simulink model "StewartPlatformSimulation"  (R2022b)
settings: Solver=VariableStepAuto  StartTime=0.0  StopTime=TF  FixedStep=stepSize  RelTol=1e-3
values from neighbouring files (symbols this model uses):
  a = s * armLegRatio    [StewartPlatformEqs.m]    (also in StewartPlatformEqs_JointAngles.m; StewartPlatformEqs_alpha.m; findRangeOfMotion_disturbance.m = 2; findh0.m)
  A0 = zeros(3,6)    [runSimulation.m]
  alpha0 = ones(1,6) * servoCalc(P_default(:,1),b(:,1),sqrt(l0_squared),s,a,beta(1))    [StewartPlatformEqs.m]    (also in StewartPlatformEqs_JointAngles.m; StewartPlatformEqs_alpha.m; runSimulation.m = alpha0')
  alpha_max = servoCenterOfRange + servoMotorRange/2    [StewartPlatformEqs.m]    (also in StewartPlatformEqs_JointAngles.m; StewartPlatformEqs_alpha.m; runSimulation.m)
  alpha_min = servoCenterOfRange - servoMotorRange/2    [StewartPlatformEqs.m]    (also in StewartPlatformEqs_JointAngles.m; StewartPlatformEqs_alpha.m; runSimulation.m)
  B = zeros(3,6)    [runSimulation.m]    (also in test.m = [0.996194698091746	0.996194698091746	-0.422618261740699	-0.5)
  beta = zeros(1,6)    [StewartPlatformEqs.m]    (also in StewartPlatformEqs_JointAngles.m; StewartPlatformEqs_alpha.m; runSimulation.m; test.m)
  defaultLegs = sqrt(l0_squared) .* ones(6,1)    [runSimulation.m]
  h0 = sqrt(l0_squared - (p(1,1) - b(1,1))^2 - (p(2,1) - b(2,1))^2) - p(3,1)    [StewartPlatformEqs.m]    (also in StewartPlatformEqs_JointAngles.m; StewartPlatformEqs_alpha.m; findROM_disturbance.m = platformParams.defaultHeight; findh0.m)
  l_max = s + a    [StewartPlatformEqs.m]    (also in StewartPlatformEqs_JointAngles.m; StewartPlatformEqs_alpha.m; runSimulation.m)
  P = circshift(P,[0 1])    [runSimulation.m]    (also in test.m = [0.458861149080837	0.458861149080837	0.338094609392560	-0.79)
  P_default = Tdefault + p    [StewartPlatformEqs.m]    (also in StewartPlatformEqs_JointAngles.m; StewartPlatformEqs_alpha.m; runSimulation.m = Tdefault + P)
  s = sqrt(legRestingLength^2 / (1+armLegRatio))    [StewartPlatformEqs.m]    (also in StewartPlatformEqs_JointAngles.m; StewartPlatformEqs_alpha.m; findh0.m; runSimulation.m = sqrt(restingLegLength^2 / (1+armLegRatio)))
settings Model: Creator=peter  LastModifiedBy=peter
settings DebuggingCC: UnderSpecifiedDimensionMsg=error

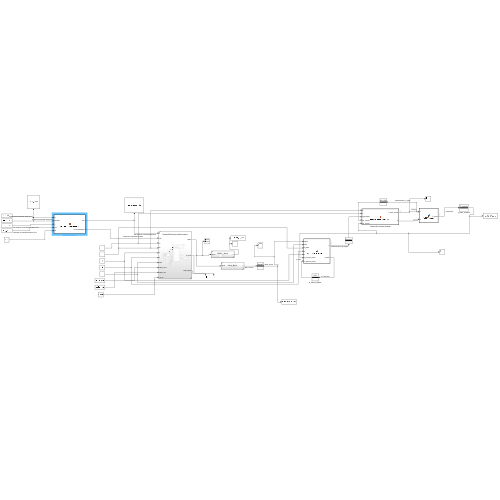
[thumbnail: Simulink's stored preview of the top-level diagram]
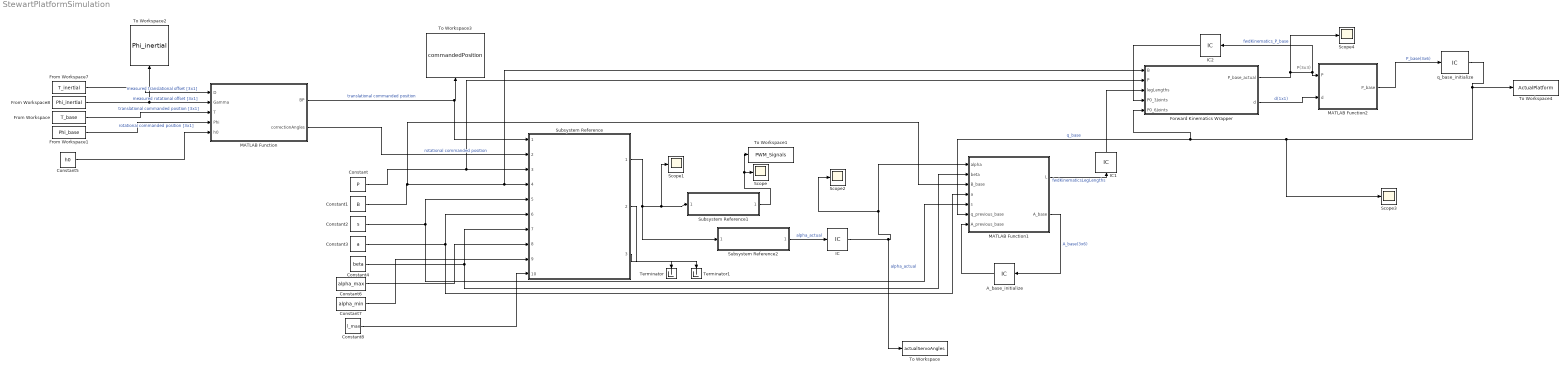
== system StewartPlatformSimulation ==
  note: P(3x3)
  A_base_initialize : InitialCondition  Value=A0
  Constant : Constant  Value=P
  Constant1 : Constant  Value=B
  Constant2 : Constant  Value=s
  Constant3 : Constant  Value=a
  Constant4 : Constant  Value=beta
  Constant5 : Constant  Value=h0
  Constant6 : Constant  Value=alpha_max
  Constant7 : Constant  Value=alpha_min
  Constant8 : Constant  Value=l_max
  Forward Kinematics Wrapper : MATLAB Function  TreatAsAtomicUnit=on
  From Workspace : FromWorkspace  VariableName=T_base
  From Workspace1 : FromWorkspace  VariableName=Phi_base
  From Workspace7 : FromWorkspace  VariableName=T_inertial
  From Workspace8 : FromWorkspace  VariableName=Phi_inertial
  IC : InitialCondition  Value=alpha0
  IC1 : InitialCondition  Value=defaultLegs
  IC2 : InitialCondition  Value=[0 0 0;0 0 0;0 0 0]
  MATLAB Function : MATLAB Function  TreatAsAtomicUnit=on
  MATLAB Function1 : MATLAB Function  TreatAsAtomicUnit=on
  MATLAB Function2 : MATLAB Function  TreatAsAtomicUnit=on
  Scope{,1..4} (5 alike) : Scope
  Subsystem Reference : Subsystem  ReferencedSubsystem=StewartPlatformInverseKinematics
  Subsystem Reference1 : Subsystem  ReferencedSubsystem=MyRio__block
  Subsystem Reference2 : Subsystem  ReferencedSubsystem=Servo_Block
  Terminator : Terminator
  Terminator1 : Terminator
  To Workspace : ToWorkspace  VariableName=actualServoAngles  SaveFormat=Timeseries  SampleTime=-1
  To Workspace1 : ToWorkspace  VariableName=PWM_Signals  SaveFormat=Timeseries  SampleTime=-1
  To Workspace2 : ToWorkspace  VariableName=Phi_inertial  SaveFormat=Timeseries  SampleTime=-1
  To Workspace3 : ToWorkspace  VariableName=commandedPosition  SaveFormat=Timeseries  SampleTime=-1
  To Workspace4 : ToWorkspace  VariableName=ActualPlatform  SaveFormat=Timeseries  SampleTime=-1
  q_base_initialize : InitialCondition  Value=P_default
  wires:
  MATLAB Function/1(BP) -> Subsystem Reference/1, To Workspace3/1  "translational commanded position"
  MATLAB Function/2(correctionAngles) -> Subsystem Reference/2  "rotational commanded position"
  Constant/1 -> Forward Kinematics Wrapper/2(P), Subsystem Reference/3
  Constant1/1 -> MATLAB Function1/3(B_base), Forward Kinematics Wrapper/1(B), Subsystem Reference/4
  Constant2/1 -> MATLAB Function1/5(s), Subsystem Reference/5
  Constant3/1 -> Subsystem Reference/6, MATLAB Function1/4(a)
  Constant4/1 -> Subsystem Reference/7, MATLAB Function1/2(beta)
  From Workspace1/1 -> MATLAB Function/4(Phi)  "rotational commanded position [3x1]"
  From Workspace/1 -> MATLAB Function/3(T)  "translational commanded position [3x1]"
  From Workspace8/1 -> MATLAB Function/2(Gamma), To Workspace2/1  "measured rotational offset [3x1]"
  From Workspace7/1 -> MATLAB Function/1(D)  "measured translational offset [3x1]"
  Subsystem Reference/1 -> Subsystem Reference2/1, Scope1/1, Subsystem Reference1/1
  Subsystem Reference1/1 -> To Workspace1/1, Scope/1
  Constant5/1 -> MATLAB Function/5(h0)
  Constant6/1 -> Subsystem Reference/8
  Constant7/1 -> Subsystem Reference/9
  Constant8/1 -> Subsystem Reference/10
  IC/1 -> To Workspace/1, Scope2/1, MATLAB Function1/1(alpha)  "alpha_actual"
  Subsystem Reference/2 -> Terminator1/1
  Subsystem Reference/3 -> Terminator/1
  MATLAB Function1/2(A_base) -> A_base_initialize/1  "A_base(3x6)"
  IC1/1 -> Forward Kinematics Wrapper/3(legLengths)
  A_base_initialize/1 -> MATLAB Function1/7(A_previous_base)
  q_base_initialize/1 -> To Workspace4/1, Scope3/1, Forward Kinematics Wrapper/5(P0_6Joints), MATLAB Function1/6(q_previous_base)  "q_base"
  Subsystem Reference2/1 -> IC/1  "alpha_actual"
  MATLAB Function2/1(P_base) -> q_base_initialize/1  "P_base(3x6)"
  Forward Kinematics Wrapper/2(d) -> MATLAB Function2/2(d)  "d(1x1)"
  Forward Kinematics Wrapper/1(P_base_actual) -> Scope4/1, IC2/1, MATLAB Function2/1(P)  "fwdKinematics_P_base"
  MATLAB Function1/1(L) -> IC1/1  "fwdKinematicsLegLengths"
  IC2/1 -> Forward Kinematics Wrapper/4(P0_3Joints)

== matlab function StewartPlatformSimulation/MATLAB Function ==
  data: D input; BP output; Gamma input; T input; Phi input; correctionAngles output; h0 input
function [BP, correctionAngles] = baseToStaticPlatformPosition(D,Gamma,T,Phi,h0)
% calculate angle offset from inertial frame
gammaX = Gamma(1) + Phi(1);
gammaY = Gamma(2) + Phi(2);
gammaZ = Gamma(3) + Phi(3);

OP = T+[0;0;h0]; % vector from origin of inertial frame (O) to origin of platform (P)

R = rotz(gammaZ)*roty(gammaY)*rotx(gammaX); % 3x3 rotation matrix

BP = D + R'*(OP - D); %BP is the base origin to platform origin vector
correctionAngles = -Gamma;
BP

== matlab function StewartPlatformSimulation/Forward Kinematics Wrapper ==
  data: B input; P_base_actual output; P input; legLengths input; d output; P0_3Joints input; P0_6Joints input
function [P_base_actual,d]  = forwardKinematicsWrapper(B,P,legLengths, P0_3Joints, P0_6Joints)

if P0_3Joints(3) ~= 0
    P_input = P0_3Joints;
else
    P_input = P0_6Joints;
end

[P_base_actual,d] = forwardKinematics(B,P,legLengths,P_input);
% P0_3Joints
% legLengths
% P_base_actual

== matlab function StewartPlatformSimulation/MATLAB Function1 ==
  data: alpha input; L output; beta input; B_base input; a input; s input; q_previous_base input; A_previous_base input; A_base output
function [L, A_base] = alpha2legLengthWrapper(alpha, beta, B_base, a, s, q_previous_base, A_previous_base)
% alpha
[L, A_base] = alpha2legLength(alpha, beta, B_base, a, s, q_previous_base, A_previous_base);
% q_previous_base
% A_previous_base
% L

== matlab function StewartPlatformSimulation/MATLAB Function2 ==
  data: P input; P_base output; d input
function P_base = find6PWrapper(P,d)
% P
P_base = find6P(P,d);
% P_base
